simulink library "arduino"  (R2016a)
settings: Solver=ode45  StartTime=0.0  StopTime=10.0  RelTol=1e-3
settings Model: Creator=maste_000  LastModifiedBy=maste_000
settings DataIOCC: LimitDataPoints=on
settings DebuggingCC: AllowSymbolicDim=off

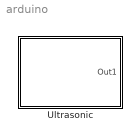
== system arduino ==
  Ultrasonic : Subsystem  mask{useInch=on, pinNum=3, SampleTime=0.1}
      mask prompts: SampleTime "Simulink:blkprm_prompts:AllSrcBlksSampleTime"
      mask TypeOptions useInch: MATLAB System/useInch
      mask TypeOptions pinNum: MATLAB System/pinNum
      mask TypeOptions SampleTime: Constant/SampleTime
      mask Display: image('download (1).jpg');

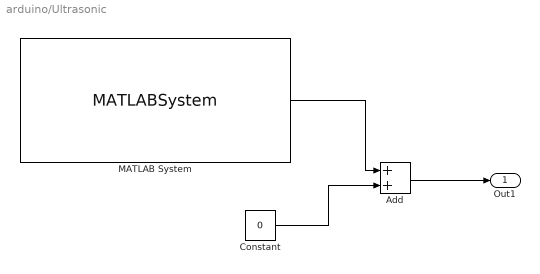
== system arduino/Ultrasonic ==
  Add : Sum
  Constant : Constant  Value=0  SampleTime=SampleTime
  MATLAB System : MATLABSystem  System=arduino.USSensor  useInch=on  pinNum=pinNum  SimulateUsing=Interpreted execution
      mask Type: arduino.USSensor
      mask Display:
      | disp('USSensor');
      | port_label('output',1,'recordedDistance');
  Out1 : Outport
  wires:
  Constant/1 -> Add/2
  Add/1 -> Out1/1
  MATLAB System/1 -> Add/1
